simulink model "Quadcopter_V3"  (R2024a)
settings: Solver=ode4  StartTime=0.0  StopTime=inf  FixedStep=0.01  RelTol=1e-3
libraries: aerolibpropulsion2 x4, slpidlib x1, shared6dof x1, sharedtransform x1, aerolibatmos2 x1, aerolibanimutils x1, uavutilslib x1
settings Model: Creator=aceco  LastModifiedBy=aceco

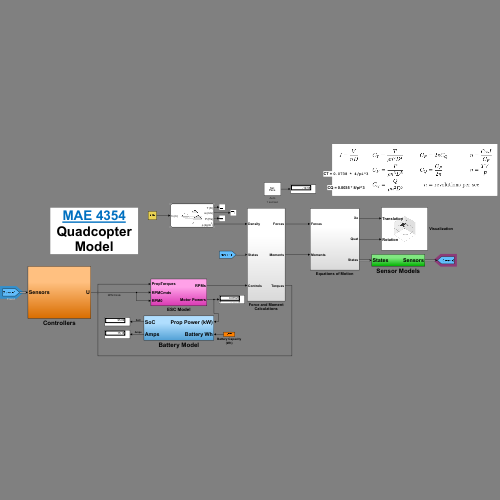
[thumbnail: Simulink's stored preview of the top-level diagram]
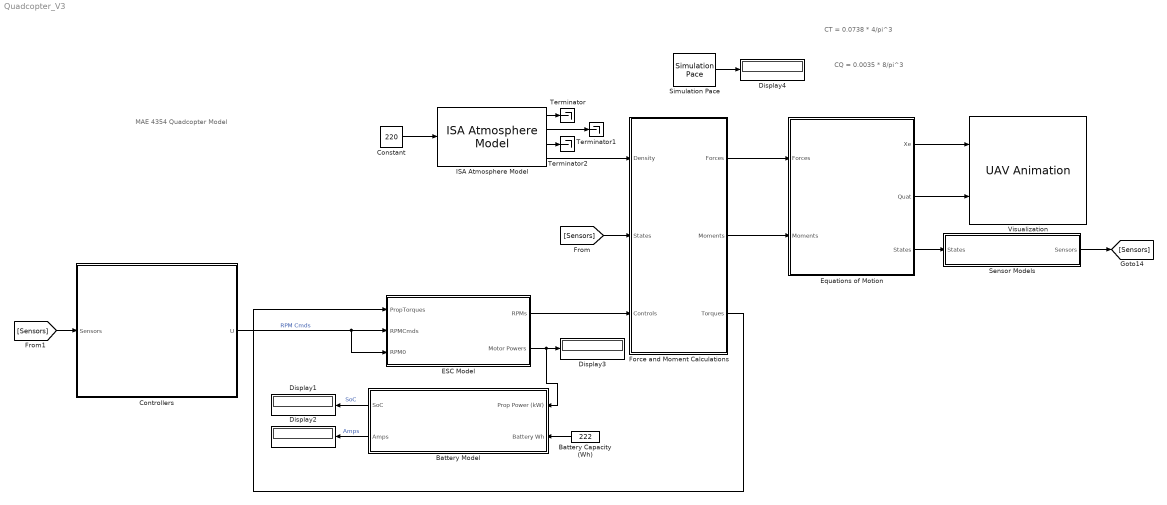
== system Quadcopter_V3 ==
  note: CQ = 0.0035 * 8/pi^3
  note: CT = 0.0738 * 4/pi^3
  note: MAE 4354
      | Quadcopter Model
  Battery Capacity (Wh) : Constant  Value=222
  Battery Model : Subsystem
  Constant : Constant  Value=220
  Controllers : Subsystem
  Display{1..4} (4 alike) : Display
  ESC Model : Subsystem
  Equations of Motion : Subsystem
  Force and Moment Calculations : Subsystem
  ISA Atmosphere Model : aerolibatmos2/ISA Atmosphere Model  useExtended=off  action=Warning  custom=off  viscosityOut=off  g=9.80665  gamma=1.4  R=287.0531  L=0.0065  h_trop=11000  h_strat=20000  rho0=1.225  P0=101325  T0=288.15  h0=0  S=110.4  Tref=273.15  muref=1.716e-5
  Sensor Models : Subsystem
  Simulation Pace : aerolibanimutils/Simulation Pace  SimulationPace=1  SleepMode=Auto  OutputPaceError=on  SampleTime=-1
  Terminator : Terminator
  Terminator1 : Terminator
  Terminator2 : Terminator
  Visualization : uavutilslib/UAV Animation  UAVType=Multirotor  UAVSize=1  InertialZDirection=Down  SampleTime=-1
  wires:
  ISA Atmosphere Model/1 -> Terminator/1
  ISA Atmosphere Model/2 -> Terminator1/1
  ISA Atmosphere Model/3 -> Terminator2/1
  Constant/1 -> ISA Atmosphere Model/1
  Simulation Pace/1 -> Display4/1
  Equations of Motion/1(Xe) -> Visualization/1
  Equations of Motion/2(Quat) -> Visualization/2
  Equations of Motion/3(States) -> Sensor Models/1(States)
  ISA Atmosphere Model/4 -> Force and Moment Calculations/1(Density)
  Force and Moment Calculations/1(Forces) -> Equations of Motion/1(Forces)
  Force and Moment Calculations/2(Moments) -> Equations of Motion/2(Moments)
  [Sensors] -> Force and Moment Calculations/2(States)
  ESC Model/1(RPMs) -> Force and Moment Calculations/3(Controls)
  Controllers/1(U) -> ESC Model/3(RPM0), ESC Model/2(RPMCmds)  "RPM Cmds"
  Force and Moment Calculations/3(Torques) -> ESC Model/1(PropTorques)
  Battery Model/2(Amps) -> Display2/1  "Amps"
  Battery Model/1(SoC) -> Display1/1  "SoC"
  Battery Capacity (Wh)/1 -> Battery Model/2(Battery Wh)
  ESC Model/2(Motor Powers) -> Battery Model/1(Prop Power (kW)), Display3/1
  Sensor Models/1(Sensors) -> [Sensors]
  [Sensors] -> Controllers/1(Sensors)

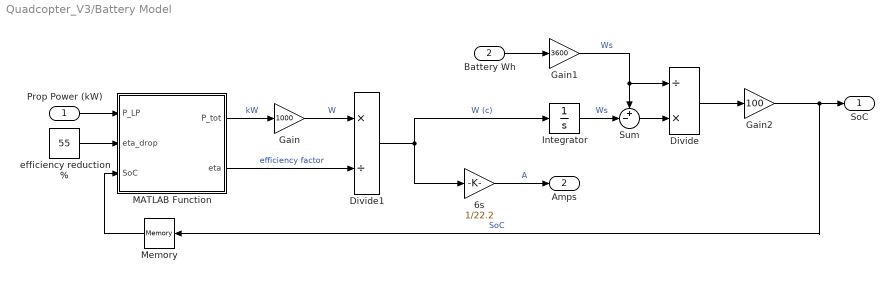
== system Quadcopter_V3/Battery Model ==
  Prop Power (kW) : Inport
  Battery Wh : Inport  Port=2
  6s : Gain  Gain=1/22.2
  Divide : Product  Inputs=/*
  Divide1 : Product  Inputs=*/
  Gain : Gain  Gain=1000
  Gain1 : Gain  Gain=3600
  Gain2 : Gain  Gain=100
  Integrator : Integrator
  MATLAB Function : MATLAB Function  TreatAsAtomicUnit=on
  Memory : Memory  InitialCondition=100
  Sum : Sum  Inputs=+-|
  efficiency reduction % : Constant  Value=55
  SoC : Outport
  Amps : Outport  Port=2
  wires:
  Battery Wh/1 -> Gain1/1
  6s/1 -> Amps/1  "A"
  Prop Power (kW)/1 -> MATLAB Function/1(P_LP)
  MATLAB Function/1(P_tot) -> Gain/1  "kW"
  Sum/1 -> Divide/2
  Integrator/1 -> Sum/2  "Ws"
  Divide/1 -> Gain2/1
  Gain2/1 -> Memory/1, SoC/1  "SoC"
  Divide1/1 -> 6s/1, Integrator/1  "W (c)"
  Gain1/1 -> Sum/1, Divide/1  "Ws"
  Gain/1 -> Divide1/1  "W"
  MATLAB Function/2(eta) -> Divide1/2  "efficiency factor"
  Memory/1 -> MATLAB Function/3(SoC)
  efficiency reduction %/1 -> MATLAB Function/2(eta_drop)

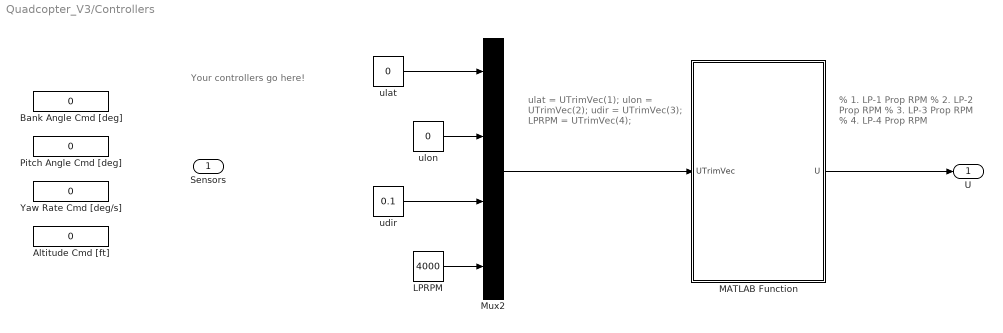
== system Quadcopter_V3/Controllers ==
  note: Your controllers go here!
  note: ulat = UTrimVec(1);
      | ulon = UTrimVec(2);
      | udir = UTrimVec(3);
      | LPRPM = UTrimVec(4);
  note: % 1. LP-1 Prop RPM
      | % 2. LP-2 Prop RPM
      | % 3. LP-3 Prop RPM
      | % 4. LP-4 Prop RPM
  Sensors : Inport
  Altitude Cmd [ft] : Constant  Value=0
  Bank Angle Cmd [deg] : Constant  Value=0
  LPRPM : Constant  Value=4000
  MATLAB Function : MATLAB Function  TreatAsAtomicUnit=on
  Mux2 : Mux
  Pitch Angle Cmd [deg] : Constant  Value=0
  Yaw Rate Cmd [deg/s] : Constant  Value=0
  udir : Constant  Value=0.1
  ulat : Constant  Value=0
  ulon : Constant  Value=0
  U : Outport
  wires:
  ulat/1 -> Mux2/1
  ulon/1 -> Mux2/2
  Mux2/1 -> MATLAB Function/1(UTrimVec)
  LPRPM/1 -> Mux2/4
  udir/1 -> Mux2/3
  MATLAB Function/1(U) -> U/1

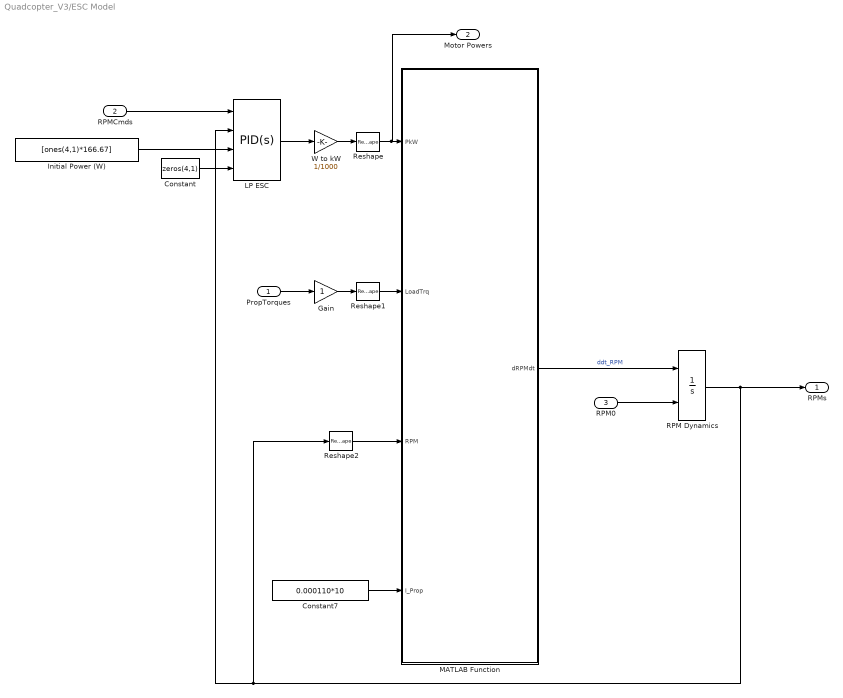
== system Quadcopter_V3/ESC Model ==
  PropTorques : Inport
  RPMCmds : Inport  Port=2
  RPM0 : Inport  Port=3
  Constant : Constant  Value=zeros(4,1)
  Constant7 : Constant  Value=0.000110*10
  Gain : Gain
  Initial Power (W) : Constant  Value=[ones(4,1)*166.67]
  LP ESC : slpidlib/PID Controller (2DOF)  Controller=PID  Form=Parallel  TimeDomain=Continuous-time  UseExternalTs=off  SampleTime=-1  IntegratorMethod=Forward Euler  FilterMethod=Forward Euler  ControllerParametersSource=internal  P=2  I=3  UseKiTs=off  D=0  UseExternalDerivativeSource=off  N=100  UseFilter=on  b=1  c=0  TunerSelectOption=Transfer Function Based (PID Tuner App)  InitialConditionSource=external  InitialConditionForIntegrator=0  InitialConditionForFilter=0  DifferentiatorICPrevScaledInput=0  ExternalReset=none  TrackingMode=off  Kt=1  LimitOutput=on  SatLimitsSource=internal  UpperSaturationLimit=300  LowerSaturationLimit=-300  LinearizeAsGain=on  AntiWindupMode=clamping  Kb=1  LimitIntegrator=off  UpperIntegratorSaturationLimit=inf  LowerIntegratorSaturationLimit=-inf  POutMin=[]  POutMax=[]  IOutMin=[]  IOutMax=[]  DOutMin=[]  DOutMax=[]  NOutMin=[]  NOutMax=[]  bOutMin=[]  bOutMax=[]  cOutMin=[]  cOutMax=[]  SumOutMin=[]  SumOutMax=[]  SaturationOutMin=[]  SaturationOutMax=[]  PParamMin=[]  PParamMax=[]  IParamMin=[]  IParamMax=[]  DParamMin=[]  DParamMax=[]  NParamMin=[]  NParamMax=[]  bParamMin=[]  bParamMax=[]  cParamMin=[]  cParamMax=[]  KbParamMin=[]  KbParamMax=[]  KtParamMin=[]  KtParamMax=[]  KbOutMin=[]  KbOutMax=[]  KtOutMin=[]  KtOutMax=[]  IntegratorOutMin=[]  IntegratorOutMax=[]  FilterOutMin=[]  FilterOutMax=[]  SumI1OutMin=[]  SumI1OutMax=[]  SumI2OutMin=[]  SumI2OutMax=[]  SumI3OutMin=[]  SumI3OutMax=[]  SumI4OutMin=[]  SumI4OutMax=[]  SumDOutMin=[]  SumDOutMax=[]  Sum1OutMin=[]  Sum1OutMax=[]  Sum2OutMin=[]  Sum2OutMax=[]  Sum3OutMin=[]  Sum3OutMax=[]  DifferentiatorOutMin=[]  DifferentiatorOutMax=[]  FilterDiffOutCoefMin=[]  FilterDiffOutCoefMax=[]  ReciprocalOutMin=[]  ReciprocalOutMax=[]  SumDenOutMin=[]  SumDenOutMax=[]  SumNumOutMin=[]  SumNumOutMax=[]  DivideOutMin=[]  DivideOutMax=[]  UdiffTsProdOutMin=[]  UdiffTsProdOutMax=[]  NTsProdOutMin=[]  NTsProdOutMax=[]  UintegralTsProdOutMin=[]  UintegralTsProdOutMax=[]  UngainTsProdOutMin=[]  UngainTsProdOutMax=[]  ClampingZeroOutDataTypeStr=Inherit: Inherit via back propagation  ClampingZeroOutMin=[]  ClampingZeroOutMax=[]  FilterDenConstantOutDataTypeStr=Inherit: Inherit via back propagation  FilterDenConstantOutMin=[]  FilterDenConstantOutMax=[]  PCopyOutDataTypeStr=Inherit: Inherit via back propagation  PCopyOutMin=[]  PCopyOutMax=[]  NCopyOutDataTypeStr=Inherit: Inherit via back propagation  NCopyOutMin=[]  NCopyOutMax=[]  IntegratorContinuousStateAttributes=''  IntegratorStateMustResolveToSignalObject=off  IntegratorRTWStateStorageClass=Auto  FilterContinuousStateAttributes=''  FilterStateMustResolveToSignalObject=off  FilterRTWStateStorageClass=Auto  ParallelPVariant=InternalParameters  IdealPVariant=Disabled  IVariant=InternalParameters  DVariant=InternalParameters  bVariant=InternalParameters  cVariant=InternalParameters  IntegratorVariant=Continuous  SatVariant=Enabled  AWVariant=ContClampingParallel  PCopyVariant=Disabled  TRVariant=Disabled  FdbkBlocksVariant=Forward  IdealPFdbkVariant=Disabled  SatFdbkVariant=Disabled  DerivativeFilterVariant=ContFilter  NVariant=InternalParameters  NCopyVariant=Disabled  FilterICVariant=ExternalICs  IntegratorICVariant=ExternalICs  ExternalResetVariant=Disabled  TRSumVariant=Passthrough  SumFdbkVariant=Disabled  SumVariant=Sum_PID  TsampFilterVariant=InternalTs  TsampNgainVariant=Passthrough  TsampIntegralVariant=Disabled_SignalSpec  ExternalSaturationOutDataTypeStr=Inherit: Same as second input  DerivativeSourceVariant=ErrorSignal
  MATLAB Function : MATLAB Function  TreatAsAtomicUnit=on
  RPM Dynamics : Integrator  InitialConditionSource=external  LimitOutput=on  UpperSaturationLimit=12000  LowerSaturationLimit=0
  Reshape : Reshape  OutputDimensionality=Row vector (2-D)
  Reshape1 : Reshape  OutputDimensionality=Row vector (2-D)
  Reshape2 : Reshape  OutputDimensionality=Column vector (2-D)
  W to kW : Gain  Gain=1/1000
  RPMs : Outport
  Motor Powers : Outport  Port=2
  wires:
  RPM0/1 -> RPM Dynamics/2
  MATLAB Function/1(dRPMdt) -> RPM Dynamics/1  "ddt_RPM"
  RPM Dynamics/1 -> RPMs/1, LP ESC/2, Reshape2/1
  Constant/1 -> LP ESC/4
  Constant7/1 -> MATLAB Function/4(I_Prop)
  Reshape/1 -> Motor Powers/1, MATLAB Function/1(PkW)
  Reshape1/1 -> MATLAB Function/2(LoadTrq)
  LP ESC/1 -> W to kW/1
  Reshape2/1 -> MATLAB Function/3(RPM)
  PropTorques/1 -> Gain/1
  W to kW/1 -> Reshape/1
  Initial Power (W)/1 -> LP ESC/3
  RPMCmds/1 -> LP ESC/1
  Gain/1 -> Reshape1/1

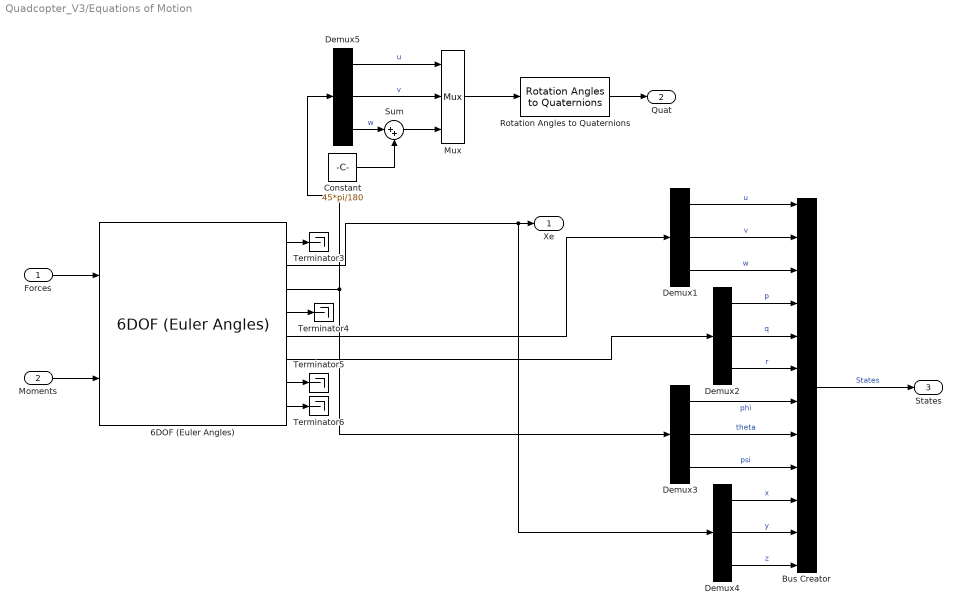
== system Quadcopter_V3/Equations of Motion ==
  Forces : Inport
  Moments : Inport  Port=2
  6DOF (Euler Angles) : shared6dof/6DOF (Euler Angles)  units=Metric (MKS)  mtype=Fixed  rep=Euler Angles  xme_0=[0 0 0]  Vm_0=[0 0 0]  eul_0=[0 0 0]  pm_0=[0 0 0]  mass_0=6.8  mass_e=0.5  mass_f=2.0  inertia=eye(3)  inertia_e=eye(3)  inertia_f=2*eye(3)  k_quat=1.0  vre_flag=on  abi_flag=off  aMode=0  xme_statename=''  Vm_statename=''  eul_statename=''  quat_statename=''  pm_statename=''  mass_statename=''
  Bus Creator : BusCreator  Inputs=12
  Constant : Constant  Value=45*pi/180
  Demux{1..5} (5 alike) : Demux  Outputs=3
  Mux : Mux  Inputs=3
  Rotation Angles to Quaternions : sharedtransform/Rotation Angles to Quaternions  rotationOrder=XYZ  aMode=aMode
  Sum : Sum  Inputs=|++
  Terminator{3..6} (4 alike) : Terminator
  Xe : Outport
  Quat : Outport  Port=2
  States : Outport  Port=3
  wires:
  Demux2/2 -> Bus Creator/5  "q"
  6DOF (Euler Angles)/3 -> Demux5/1, Demux3/1
  6DOF (Euler Angles)/2 -> Xe/1, Demux4/1
  6DOF (Euler Angles)/5 -> Demux1/1
  6DOF (Euler Angles)/7 -> Terminator5/1
  6DOF (Euler Angles)/1 -> Terminator3/1
  Demux1/1 -> Bus Creator/1  "u"
  Demux2/1 -> Bus Creator/4  "p"
  Demux4/1 -> Bus Creator/10  "x"
  Demux4/3 -> Bus Creator/12  "z"
  Demux2/3 -> Bus Creator/6  "r"
  Moments/1 -> 6DOF (Euler Angles)/2
  Demux3/2 -> Bus Creator/8  "theta"
  Demux1/2 -> Bus Creator/2  "v"
  Demux3/1 -> Bus Creator/7  "phi"
  Demux1/3 -> Bus Creator/3  "w"
  Demux3/3 -> Bus Creator/9  "psi"
  6DOF (Euler Angles)/6 -> Demux2/1
  Demux4/2 -> Bus Creator/11  "y"
  6DOF (Euler Angles)/8 -> Terminator6/1
  6DOF (Euler Angles)/4 -> Terminator4/1
  Bus Creator/1 -> States/1  "States"
  Forces/1 -> 6DOF (Euler Angles)/1
  Rotation Angles to Quaternions/1 -> Quat/1
  Demux5/1 -> Mux/1  "u"
  Demux5/2 -> Mux/2  "v"
  Demux5/3 -> Sum/1  "w"
  Sum/1 -> Mux/3
  Constant/1 -> Sum/2
  Mux/1 -> Rotation Angles to Quaternions/1

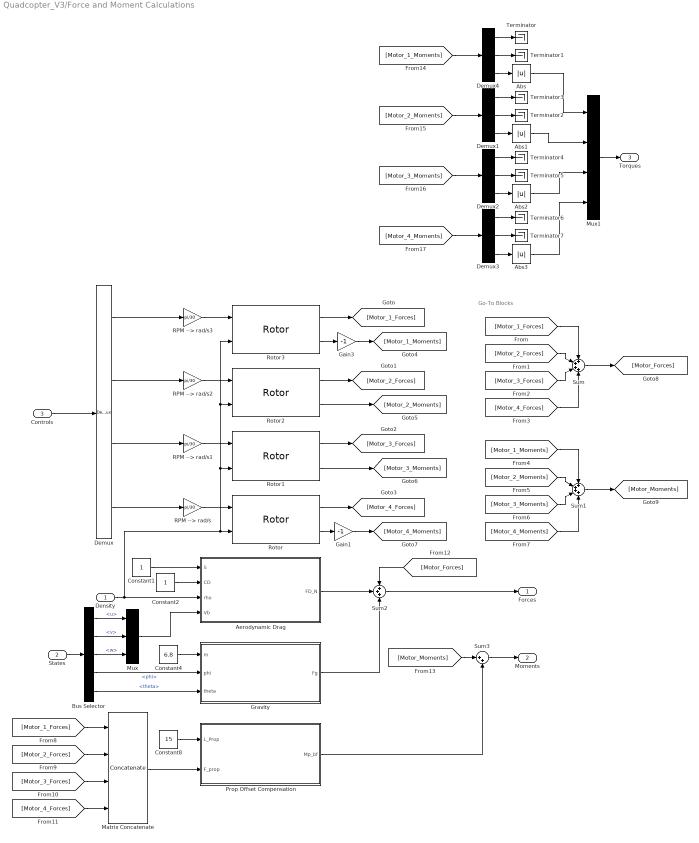
== system Quadcopter_V3/Force and Moment Calculations ==
  note: Go-To Blocks
  Density : Inport
  States : Inport  Port=2
  Controls : Inport  Port=3
  Abs{,1..3} (4 alike) : Abs  SaturateOnIntegerOverflow=off
  Aerodynamic Drag : MATLAB Function  TreatAsAtomicUnit=on
  Bus Selector : BusSelector  OutputSignals=u,v,w,phi,theta
  Constant1 : Constant
  Constant2 : Constant
  Constant4 : Constant  Value=6.8
  Constant8 : Constant  Value=15
  Demux : Demux
  Demux{1..4} (4 alike) : Demux  Outputs=3
  Gain1 : Gain  Gain=-1
  Gain3 : Gain  Gain=-1
  Gravity : MATLAB Function  TreatAsAtomicUnit=on
  Matrix Concatenate : Concatenate  NumInputs=4  Mode=Multidimensional array  ConcatenateDimension=2
  Mux : Mux  Inputs=3
  Mux1 : Mux
  Prop Offset Compensation : MATLAB Function  TreatAsAtomicUnit=on
  RPM --> rad/s{,1..3} (4 alike) : Gain  Gain=pi/30
  Rotor{,1..3} (4 alike) : aerolibpropulsion2/Rotor  units=Metric (MKS)  modelMode=Without flap effects  blockSelect=Single  config=Quadcopter X  Nr=1  l=0.0624  h=-0.0159  Arm=[0;0;0]  Nb=2  CTcheck=off  CT=0.0738 * 4/pi^3  CQ=0.0035 * 8/pi^3  CTout=off  R=15/39.37/2  c=0.0080  e=0  clalpha=5.5  gamma=0.6051  twistType=Linear  theta0=0.2548  theta1=-0.1361  thetaTip=0.1018  Vb=[0;0;0]  pqr=[0;0;0]
      settings: LibrarySourceBlock=aerolibrotor/Rotor
  Sum : Sum  Inputs=++++
  Sum1 : Sum  Inputs=++++
  Sum2 : Sum  Inputs=+++
  Sum3 : Sum  Inputs=|++
  Terminator{,1..7} (8 alike) : Terminator
  Forces : Outport
  Moments : Outport  Port=2
  Torques : Outport  Port=3
  wires:
  RPM --> rad/s3/1 -> Rotor3/1
  Constant4/1 -> Gravity/1(m)
  Constant1/1 -> Aerodynamic Drag/1(S)
  Rotor3/1 -> [Motor_1_Forces]
  RPM --> rad/s/1 -> Rotor/1
  [Motor_Forces] -> Sum2/1
  Sum/1 -> [Motor_Forces]
  RPM --> rad/s2/1 -> Rotor2/1
  Rotor/1 -> [Motor_4_Forces]
  [Motor_2_Forces] -> Sum/2
  Gain3/1 -> [Motor_1_Moments]
  [Motor_3_Forces] -> Sum/3
  Rotor1/2 -> [Motor_3_Moments]
  Rotor1/1 -> [Motor_3_Forces]
  [Motor_4_Forces] -> Sum/4
  Rotor2/1 -> [Motor_2_Forces]
  Rotor2/2 -> [Motor_2_Moments]
  Constant8/1 -> Prop Offset Compensation/1(L_Prop)
  Density/1 -> Aerodynamic Drag/3(rho), Rotor3/2, Rotor2/2, Rotor1/2, Rotor/2
  Matrix Concatenate/1 -> Prop Offset Compensation/2(F_prop)
  Rotor3/2 -> Gain3/1
  [Motor_4_Moments] -> Sum1/4
  Mux/1 -> Aerodynamic Drag/4(Vb)
  Sum3/1 -> Moments/1
  RPM --> rad/s1/1 -> Rotor1/1
  [Motor_1_Forces] -> Matrix Concatenate/1
  [Motor_3_Forces] -> Matrix Concatenate/3
  [Motor_1_Moments] -> Sum1/1
  Gain1/1 -> [Motor_4_Moments]
  [Motor_3_Moments] -> Sum1/3
  Aerodynamic Drag/1(FD_N) -> Sum2/2
  [Motor_2_Moments] -> Sum1/2
  [Motor_4_Forces] -> Matrix Concatenate/4
  [Motor_1_Forces] -> Sum/1
  [Motor_2_Forces] -> Matrix Concatenate/2
  Sum1/1 -> [Motor_Moments]
  Constant2/1 -> Aerodynamic Drag/2(CD)
  Prop Offset Compensation/1(Mp_bf) -> Sum3/2
  Rotor/2 -> Gain1/1
  Gravity/1(Fg) -> Sum2/3
  [Motor_Moments] -> Sum3/1
  Sum2/1 -> Forces/1
  States/1 -> Bus Selector/1
  Bus Selector/5 -> Gravity/3(theta)  "<theta>"
  Bus Selector/4 -> Gravity/2(phi)  "<phi>"
  Bus Selector/1 -> Mux/1  "<u>"
  Bus Selector/2 -> Mux/2  "<v>"
  Bus Selector/3 -> Mux/3  "<w>"
  Demux/4 -> RPM --> rad/s/1
  Demux/3 -> RPM --> rad/s1/1
  Demux/2 -> RPM --> rad/s2/1
  Demux/1 -> RPM --> rad/s3/1
  Controls/1 -> Demux/1
  [Motor_1_Moments] -> Demux4/1
  [Motor_2_Moments] -> Demux1/1
  [Motor_3_Moments] -> Demux2/1
  [Motor_4_Moments] -> Demux3/1
  Demux4/1 -> Terminator/1
  Demux4/2 -> Terminator1/1
  Demux1/2 -> Terminator2/1
  Demux1/1 -> Terminator3/1
  Demux2/1 -> Terminator4/1
  Demux2/2 -> Terminator5/1
  Demux3/1 -> Terminator6/1
  Demux3/2 -> Terminator7/1
  Demux4/3 -> Abs/1
  Demux1/3 -> Abs1/1
  Demux3/3 -> Abs3/1
  Demux2/3 -> Abs2/1
  Abs/1 -> Mux1/1
  Abs1/1 -> Mux1/2
  Abs2/1 -> Mux1/3
  Abs3/1 -> Mux1/4
  Mux1/1 -> Torques/1

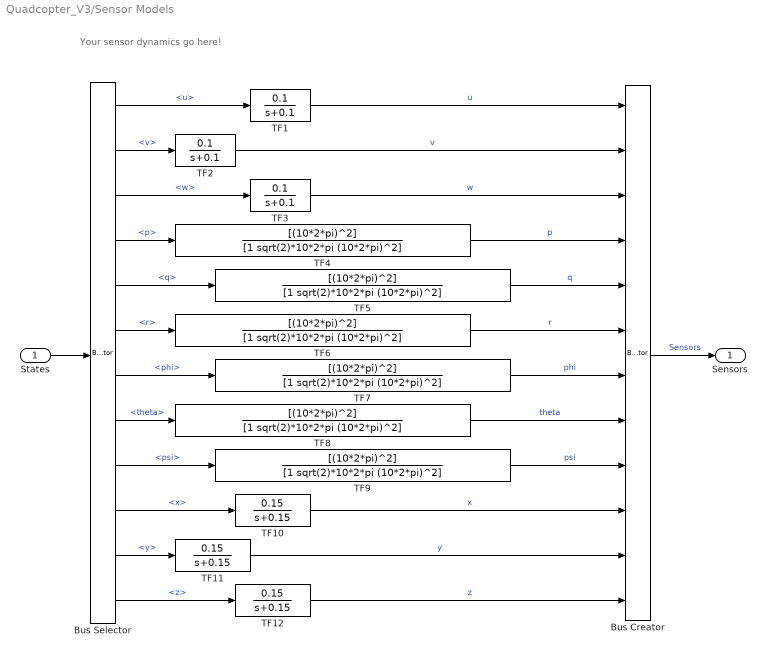
== system Quadcopter_V3/Sensor Models ==
  note: Your sensor dynamics go here!
  States : Inport
  Bus Creator : BusCreator  Inputs=12
  Bus Selector : BusSelector  OutputSignals=u,v,w,p,q,r,phi,theta,psi,x,y,z
  TF1 : TransferFcn  Numerator=[0.1]  Denominator=[1 0.1]
  TF10 : TransferFcn  Numerator=[0.15]  Denominator=[1 0.15]
  TF11 : TransferFcn  Numerator=[0.15]  Denominator=[1 0.15]
  TF12 : TransferFcn  Numerator=[0.15]  Denominator=[1 0.15]
  TF2 : TransferFcn  Numerator=[0.1]  Denominator=[1 0.1]
  TF3 : TransferFcn  Numerator=[0.1]  Denominator=[1 0.1]
  TF{4..9} (6 alike) : TransferFcn  Numerator=[(10*2*pi)^2]  Denominator=[1 sqrt(2)*10*2*pi (10*2*pi)^2]
  Sensors : Outport
  wires:
  States/1 -> Bus Selector/1
  Bus Selector/1 -> TF1/1  "<u>"
  Bus Selector/2 -> TF2/1  "<v>"
  Bus Selector/3 -> TF3/1  "<w>"
  Bus Selector/4 -> TF4/1  "<p>"
  Bus Selector/5 -> TF5/1  "<q>"
  Bus Selector/6 -> TF6/1  "<r>"
  Bus Selector/7 -> TF7/1  "<phi>"
  Bus Selector/8 -> TF8/1  "<theta>"
  Bus Selector/9 -> TF9/1  "<psi>"
  Bus Selector/10 -> TF10/1  "<x>"
  Bus Selector/11 -> TF11/1  "<y>"
  Bus Selector/12 -> TF12/1  "<z>"
  TF10/1 -> Bus Creator/10  "x"
  TF1/1 -> Bus Creator/1  "u"
  TF6/1 -> Bus Creator/6  "r"
  TF2/1 -> Bus Creator/2  "v"
  TF8/1 -> Bus Creator/8  "theta"
  TF11/1 -> Bus Creator/11  "y"
  TF9/1 -> Bus Creator/9  "psi"
  TF7/1 -> Bus Creator/7  "phi"
  TF3/1 -> Bus Creator/3  "w"
  TF5/1 -> Bus Creator/5  "q"
  TF12/1 -> Bus Creator/12  "z"
  TF4/1 -> Bus Creator/4  "p"
  Bus Creator/1 -> Sensors/1  "Sensors"

== matlab function Quadcopter_V3/Force and Moment Calculations/Gravity ==
  data: m input; Fg output; phi input; theta input
function Fg = fcn(m,phi,theta)
% Gravity Model in Body Axes (3-2-1 Euler, NED convention)
%
% Inputs:
%   phi   - roll angle [rad]
%   theta - pitch angle [rad]
%
% Outputs:
%   gB    - 3x1 gravity acceleration vector in body axes [m/s^2]
%
% Notes:
%   This assumes the common aerospace convention:
%     body axes: x forward, y right, z down
%     navigation frame: NED (down positive)
%   If you need gravity *force* in body axes, use: FG = m * gB
%

% initialize outputs
Fg = zeros(3,1);

% constant gravity
g = 9.80665; % [m/s^2]

% components of gravity expressed in body axes
gx = -m * g * sin(theta);
gy =  m * g * sin(phi) * cos(theta);
gz =  m * g * cos(phi) * cos(theta);

% combine into a single output
Fg = [...
    gx;
    gy;
    gz];

end

== matlab function Quadcopter_V3/Force and Moment Calculations/Aerodynamic Drag ==
  data: S input; FD_N output; CD input; rho input; Vb input
function FD_N = fcn(S,CD,rho,Vb)
% Simple Aerodynamic Drag Model
%
% Inputs:
%   S   - reference area [m^2]
%   CD  - drag coefficient [-]
%   rho - air density [kg/m^3]
%   Vb  - body-fixed velocity vector [u; v; w] [m/s]
%
% Outputs:
%   FD         - 3x1 drag force vector in body axes [N]
%

% initialize outputs
FD_N = zeros(3,1);

% split incoming velocity vector into 3 directions:
u = Vb(1);
v = Vb(2);
w = Vb(3);

% compute drag on each axis
Fx = -1/2 * rho * S * CD * abs(u) * u;
Fy = -1/2 * rho * S * CD * abs(v) * v;
Fz = -1/2 * rho * S * CD * abs(w) * w;

% combine into a single output
FD_N = [...
    Fx;
    Fy;
    Fz];

end

== matlab function Quadcopter_V3/Force and Moment Calculations/Prop Offset Compensation ==
  data: L_Prop input; Mp_bf output; F_prop input
function Mp_bf = fcn(L_Prop,F_prop)

% initialize outputs
Mp_bf = zeros(3,1);

% grab out necessary data
Fp_bfx = F_prop(1,:)';
Fp_bfy = F_prop(2,:)';
Fp_bfz = F_prop(3,:)';

% motor hub locations (n x 1)
R = ones(4,1)*L_Prop/39.37; % R" drone arm length [m]
ps_A = [135;45;225;315]; % arm angles (from 0 --> along y axis)
x_props = R.*sind(ps_A);
y_props = R.*cosd(ps_A);
z_props = (ones(4,1) + 3)/39.37; % assume CG is below (+z) motor hubs
Prop_Loc = [x_props,y_props,z_props];

% resolve these forces into body-fixed moments (r x F expansion)
Mp_bfx = y_props.*Fp_bfz - z_props.*Fp_bfy;
Mp_bfy = z_props.*Fp_bfx - x_props.*Fp_bfz;
Mp_bfz = x_props.*Fp_bfy - y_props.*Fp_bfx;

% add across all props
Mp_x = sum(Mp_bfx);
Mp_y = sum(Mp_bfy);
Mp_z = sum(Mp_bfz);

% conactenate
Mp_bf = [...
    Mp_x;
    Mp_y;
    Mp_z];

end

== matlab function Quadcopter_V3/ESC Model/MATLAB Function ==
  data: PkW input; LoadTrq input; RPM input; I_Prop input; dRPMdt output
function dRPMdt  = MotorDynamics_MP(PkW,LoadTrq,RPM,I_Prop)

%% Initializations
nProp = 4;
Q = zeros(nProp,1);
dwdt = zeros(nProp,1);
dRPMdt = zeros(nProp,1);

% max torque
Qmax = 1.5; % Nm

%% Incoming Values
PropTorque = LoadTrq';
P_in = PkW'*1000;

% prop speed in rad/s
w = RPM*2*pi/60;

%% Standard Method
Q = P_in./w;
% limit max torque
Q = max(-Qmax,min(Q,Qmax));

% equation of motion
dwdt = (Q - PropTorque)./I_Prop;
dRPMdt = dwdt*60/(2*pi);

end

== matlab function Quadcopter_V3/Battery Model/MATLAB Function ==
  data: P_LP input; P_tot output; eta_drop input; eta output; SoC input
function [P_tot,eta] = fcn(P_LP,eta_drop,SoC)

P_tot = sum(P_LP);
PW_tot = P_tot*1000;

% with a reduction in the state of charge, the battery becomes even less efficient
SoC_factor = 1 - 0.01*(SoC - 100);
% battery efficiency is a function of total power draw and SoC
eta = 1/100*(90 - eta_drop*SoC_factor/1000*PW_tot);
% eta should never drop below a logical value
eta = max(0.3,eta);

end

== matlab function Quadcopter_V3/Controllers/MATLAB Function ==
  data: UTrimVec input; U output
function U  = ControlAllocation(UTrimVec)
%% File Information
% ControlAllocation - control allocation function (vehicle-specific)
%
% DESCRIPTION: 
%   This is a vehicle-specific control allocation (mixer) function,
%   relating normalized lateral, longitudinal, directional, and other
%   control commands to control effector commands
%
% WRITTEN BY:
%   Anthony M. Comer
%   Oklahoma State University
%   Email: anthony.m.comer@nasa.gov
%
% HISTORY:
%   07 JUL 2025 - created and debugged, AMC
%
% ***FOR INTERNAL OSU USE ONLY***
%
%% Quadplane Control Effectors

% 1. LP-1 Prop RPM
% 2. LP-2 Prop RPM
% 3. LP-3 Prop RPM
% 4. LP-4 Prop RPM

%% UTrimVec Defintion

% 1. ulat --> normalized lateral control command [-1,+1]
% 2. ulon --> normalized longitudinal control command [-1,+1]
% 3. udir --> normalized directional control command [-1,+1]
% 4. LPRPM --> common LPRPM component [0,LPRPMmax]

%% Initializations / Settings
U = zeros(4,1); % this corresponds to the number of outputs

% differential RPM limits (to be exposed)
dN_lat = 1000;
dN_lon = 1000;
dN_dir = 2500;

%% Unpack Incoming Trim Vector

ulat = UTrimVec(1);
ulon = UTrimVec(2);
udir = UTrimVec(3);
LPRPM = UTrimVec(4);

% limit possible inputs
ulat = max(-1,min(ulat,1));
ulon = max(-1,min(ulon,1));
udir = max(-1,min(udir,1));

%% Propulsor Allocation

% compute differential RPM equivalents from incoming normalized commands
dlat = ulat*dN_lat;
dlon = ulon*dN_lon;
ddir = udir*dN_dir;

% common RPM differs in forward-flight as the props shut down
LPRPM0 = LPRPM;

% propulsion mixing term
dBmat_LP = [...
    +1,+1,+1,+1;
    +1,-1,+1,-1;
    +1,+1,-1,-1;
    +1,-1,-1,+1;
    ];

% mixing matrix
% N14 = dBmat(1:4,:)*[MPRPM0;dlat*MP_roll;dlon*MP_pitch;ddir*MP_yaw];
N_LP = dBmat_LP*[LPRPM0;dlat;dlon;ddir];

% combine RPMs
N = [N_LP];

%% Form Control Effector Command Vector

U = N;

end
